simulink model "acquisition_store_crc_design"  (R2021a)
settings: Solver=FixedStepDiscrete  StartTime=0.0  StopTime=10.0  FixedStep=0.1  RelTol=1e-3  EnableMultiTasking=on
settings Model: Creator=afonso.miguel  LastModifiedBy=afonso.miguel
settings SolverCC: AlgebraicLoopSolver=TrustRegion  AutoInsertRateTranBlk=on
settings DataIOCC: LimitDataPoints=on
settings OptimizationCC: LifeSpan=inf
settings DebuggingCC: AllowSymbolicDim=off  SFUnexpectedBacktrackingDiag=warning  SFNoUnconditionalDefaultTransitionDiag=warning  SFExecutionAtInitializationDiag=none  UnderSpecifiedDimensionMsg=warning  ArithmeticOperatorsInVariantConditions=warning
settings SFSimCC: SimUseLocalCustomCode=off  CustomCodeUndefinedFunction=UseInterfaceOnly
settings RTWCC: RTWUseLocalCustomCode=off
settings CodeAppCC: StateflowObjectComments=on
settings GRTTargetCC: TargetLangStandard=C89/C90 (ANSI)
settings ConfigComp: CovMetricSettings=dw  CovSaveCumulativeToWorkspaceVar=on  CovSaveSingleToWorkspaceVar=on  CovExternalEMLEnable=off  CovSFcnEnable=off

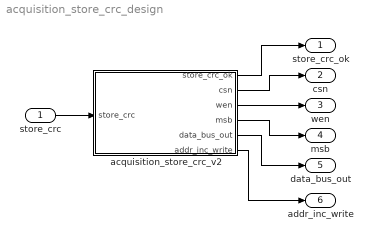
== system acquisition_store_crc_design ==
  store_crc : Inport  OutDataTypeStr=fixdt(0,1,0)
  acquisition_store_crc_v2 : Stateflow chart  TreatAsAtomicUnit=on
  store_crc_ok : Outport  OutDataTypeStr=fixdt(0,1,0)
  csn : Outport  Port=2  OutDataTypeStr=fixdt(0,1,0)
  wen : Outport  Port=3  OutDataTypeStr=fixdt(0,1,0)
  msb : Outport  Port=4  OutDataTypeStr=fixdt(0,1,0)
  data_bus_out : Outport  Port=5  OutDataTypeStr=fixdt(0,1,0)
  addr_inc_write : Outport  Port=6  OutDataTypeStr=fixdt(0,1,0)
  wires:
  store_crc/1 -> acquisition_store_crc_v2/1(store_crc)
  acquisition_store_crc_v2/1(store_crc_ok) -> store_crc_ok/1
  acquisition_store_crc_v2/2(csn) -> csn/1
  acquisition_store_crc_v2/3(wen) -> wen/1
  acquisition_store_crc_v2/4(msb) -> msb/1
  acquisition_store_crc_v2/5(data_bus_out) -> data_bus_out/1
  acquisition_store_crc_v2/6(addr_inc_write) -> addr_inc_write/1

== stateflow chart acquisition_store_crc_design/acquisition_store_crc_v2 ==
  settings: executeAtInitialization=1
  state y=wait_states [function]
    (default) -> (junction 51) : {y=3;}
  state wait_store_crc
    entry:
    csn=1;
    wen=1;
    msb=0;
    store_crc_ok=0;
    addr_inc_write=0;
  state write_lsb
    state setup_write_lsb
    state write_lsb
    state hold_write_lsb
      entry:
      addr_inc_write=1;
    setup_write_lsb -> write_lsb.write_lsb : {wen=0;
        | wait_state_counter=fi(wait_states(),0,2,0);}
    write_lsb.write_lsb -> write_lsb.write_lsb [order 1] : [wait_state_counter~=1]
        | {wait_state_counter=fi(wait_state_counter-1,0,2,0);}
    write_lsb.write_lsb -> hold_write_lsb [order 2] : {wen=1;}
  state write_msb
    state setup_write_msb
    state write_msb
    state hold_write_msb
      entry:
      addr_inc_write=1;
    setup_write_msb -> write_msb.write_msb : {wen=0;
        | wait_state_counter=fi(wait_states(),0,2,0);}
    write_msb.write_msb -> write_msb.write_msb [order 1] : [wait_state_counter~=1]
        | {wait_state_counter=fi(wait_state_counter-1,0,2,0);}
    write_msb.write_msb -> hold_write_msb [order 2] : {wen=1}
  state wait_end
  wait_store_crc -> setup_write_lsb [order 2] : {csn=0;
      | data_bus_out=1;}
  hold_write_lsb -> setup_write_msb : {msb=1;
      | addr_inc_write=0;}
  hold_write_msb -> wait_end : {store_crc_ok=1;
      | csn=1;
      | data_bus_out=0;
      | addr_inc_write=0;}
  (default) -> wait_store_crc
  wait_store_crc -> wait_store_crc [order 1] : [store_crc==0]
  wait_end -> wait_store_crc [order 1] : [store_crc==0]
  wait_end -> wait_end [order 2]
  data: y function_output; store_crc_ok output fixdt(0,1,0); store_crc input fixdt(0,1,0); csn output fixdt(0,1,0); wen output fixdt(0,1,0); msb output fixdt(0,1,0); data_bus_out output fixdt(0,1,0); wait_state_counter local fixdt(0,2,0); addr_inc_write output fixdt(0,1,0)
